simulink model "thust_block"  (R2023b)
settings: Solver=VariableStepAuto  StartTime=0.0  StopTime=10.0  RelTol=1e-3
settings Model: Creator=klyx  LastModifiedBy=klyx

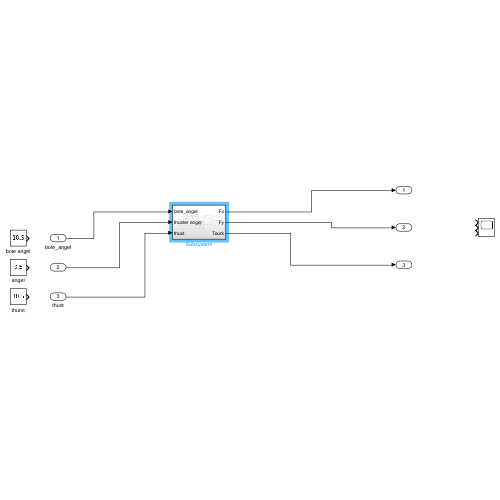
[thumbnail: Simulink's stored preview of the top-level diagram]
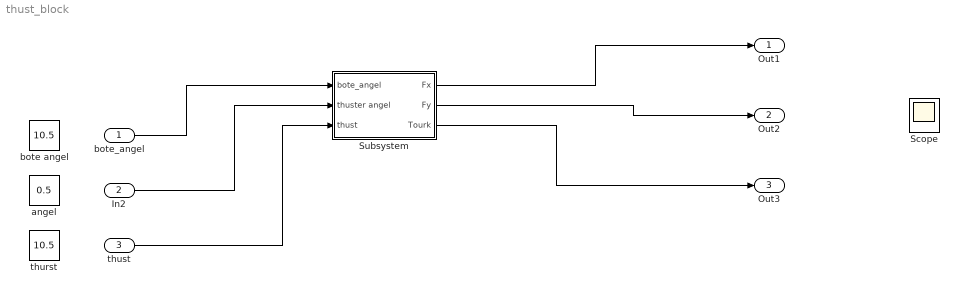
== system thust_block ==
  bote_angel : Inport
  In2 : Inport  Port=2
  thust : Inport  Port=3
  Scope : Scope  NumInputPorts=3
  Subsystem : Subsystem
  angel : Constant  Value=0.5
  bote angel : Constant  Value=10.5
  thurst : Constant  Value=10.5
  Out1 : Outport
  Out2 : Outport  Port=2
  Out3 : Outport  Port=3
  wires:
  bote_angel/1 -> Subsystem/1(bote_angel)
  In2/1 -> Subsystem/2(thuster angel)
  thust/1 -> Subsystem/3(thust)
  Subsystem/1(Fx) -> Out1/1
  Subsystem/2(Fy) -> Out2/1
  Subsystem/3(Tourk) -> Out3/1

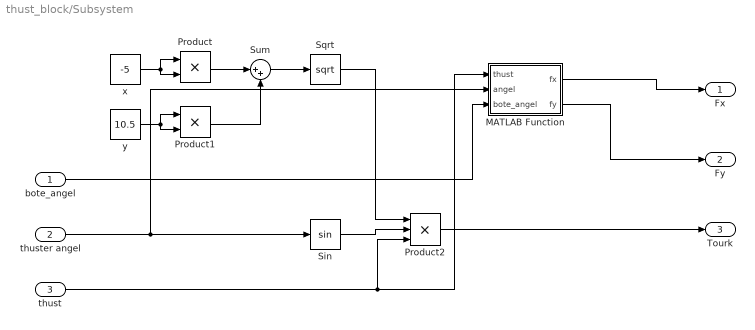
== system thust_block/Subsystem ==
  bote_angel : Inport
  thuster angel : Inport  Port=2
  thust : Inport  Port=3
  MATLAB Function : MATLAB Function  TreatAsAtomicUnit=on
  Product : Product
  Product1 : Product
  Product2 : Product  Inputs=3
  Sin : Trigonometry
  Sqrt : Sqrt
  Sum : Sum  Inputs=|++
  x : Constant  Value=-5
  y : Constant  Value=10.5
  Fx : Outport
  Fy : Outport  Port=2
  Tourk : Outport  Port=3
  wires:
  Sin/1 -> Product2/2
  Product1/1 -> Sum/2
  y/1 -> Product1/2, Product1/1
  Product/1 -> Sum/1
  thuster angel/1 -> Sin/1, MATLAB Function/2(angel)
  thust/1 -> MATLAB Function/1(thust), Product2/3
  bote_angel/1 -> MATLAB Function/3(bote_angel)
  MATLAB Function/1(fx) -> Fx/1
  MATLAB Function/2(fy) -> Fy/1
  Sum/1 -> Sqrt/1
  Product2/1 -> Tourk/1
  Sqrt/1 -> Product2/1
  x/1 -> Product/1, Product/2

== matlab function thust_block/Subsystem/MATLAB Function ==
  data: thust input; fx output; angel input; bote_angel input; fy output
function [fx,fy] = fcn(thust, angel, bote_angel)

Rx = [cos(bote_angel) -sin(bote_angel); sin(bote_angel) cos(bote_angel)];
f = [sin(angel); cos(angel)]*thust;
mf = Rx*f;
fx = mf(1);
fy = mf(2);
